simulink model "BioReator_Sfun_Tutorial"  (R2023b)
settings: Solver=VariableStepAuto  StartTime=0.0  StopTime=10.0  RelTol=1e-3
settings Model: Creator=frede  LastModifiedBy=frede

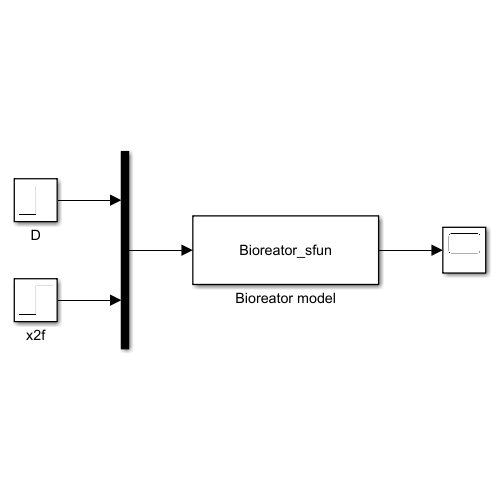
[thumbnail: Simulink's stored preview of the top-level diagram]
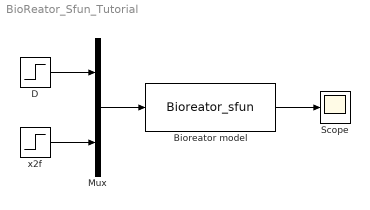
== system BioReator_Sfun_Tutorial ==
  Bioreator model : M-S-Function  FunctionName=Bioreator_sfun  Parameters=1, 1
  D : Step  Time=0  After=.4  SampleTime=0
  Mux : Mux  Inputs=2
  Scope : Scope
  x2f : Step  Time=0  After=4  SampleTime=0
  wires:
  Mux/1 -> Bioreator model/1
  x2f/1 -> Mux/2
  D/1 -> Mux/1
  Bioreator model/1 -> Scope/1
